simulink model "Thruster_Example_rw"  (R2024b)
settings: Solver=ode4  StartTime=0.0  StopTime=2000  FixedStep=0.01  RelTol=1e-3
undefined symbols (not defined in the file): Cube_L, dt, F_vec, Iws, M_rw, m_tot, norm_Ib, Omega1_init, Omega2_init, Omega3_init, Omega4_init, qb0, rad2rpm, RCS_F, RCS_F_vec, RCS_Pos, RCS_pos, RCS_PWM_Freq, RCS_Sampling_time, RCS_THR_vec, REL_TS_POS_I_0, REL_TS_VEL_I_0, RW_As, RW_Max_Speed, RW_Omegad_max, sat, SC_Ib, SC_state0, SS_Total_Mass, TC_Kepler, THR_dt, THR_Force, THR_freq, THR_Pos, TS_Ib, TS_qb0, TS_state0, TS_wb0, wb0, X, Y, Z
libraries: sm_lib x348, nesl_utility x236, simulink_extras x115, sharedtransform x64, aerolibutil x38, simulink x28, sharedutil x13
(part 16 of 16)

== matlab function Thruster_Example_rw/Prac1/Subsystem/Thruster Allocation ==
  settings: updateMethod=DISCRETE
  data: u_pwm output; F_B_cmd input; tau_B_cmd input; F_B_real output; tau_B_real output; r input; d input; F_max input
function [u_pwm, F_B_real, tau_B_real] = ALLOC_THRUSTER_PWM_16(F_B_cmd, tau_B_cmd, r, d, F_max)
%#codegen
% ============================================================
% Allocation block
% Input :
%   F_B_cmd    [3x1] desired total body force
%   tau_B_cmd  [3x1] desired total body torque
%
% Output:
%   u_pwm      [12x1] thruster duty command, 0 ~ 1
%   F_B_real   [3x1] realized body force after allocation
%   tau_B_real [3x1] realized body torque after allocation
%
% Example:
%   12-thruster layout for 6DoF control
%   Replace thruster geometry / Tmax below with your real spacecraft values.
% ============================================================

    % Build 6x12 thruster mapping matrix A
    A = build_thruster_matrix( 16, r, d, F_max);

    % Desired wrench
    w_cmd = [F_B_cmd; tau_B_cmd];

    % Bounded least-squares allocation: 0 <= u <= 1
    u_pwm = bounded_allocator_0_1(A, w_cmd);

    % Realized wrench
    w_real     = A * u_pwm;
    F_B_real   = w_real(1:3);
    tau_B_real = w_real(4:6);
end


% ============================================================
% Thruster layout
% ============================================================
function A = build_thruster_matrix(N, r, d, F_max)
    % --------------------------------------------------------
    % Example spacecraft half-size [m]
    % Replace with your real geometry
    % --------------------------------------------------------
    % L = 0.50;   % lever arm

    % --------------------------------------------------------
    % Max thrust of each thruster [N]
    % Replace with your real thruster max force
    % --------------------------------------------------------
    Tmax = F_max * ones(N,1);

    % --------------------------------------------------------
    % Thruster positions r_i in body frame [m]
    % Each column is one thruster position
    % --------------------------------------------------------
    % r = [ ...
    %      0,   0,   0,   0,   L,  -L,   L,  -L,   L,  -L,   L,  -L;
    %      L,  -L,   L,  -L,   0,   0,   0,   0,   L,   L,  -L,  -L;
    %      L,  -L,  -L,   L,   L,  -L,  -L,   L,   0,   0,   0,   0 ];

    % --------------------------------------------------------
    % Thruster unit directions d_i in body frame
    %
    % T1,T2 : +X
    % T3,T4 : -X
    % T5,T6 : +Y
    % T7,T8 : -Y
    % T9,T10: +Z
    % T11,T12:-Z
    % --------------------------------------------------------
    % d = [ ...
    %      1,   1,  -1,  -1,   0,   0,   0,   0,   0,   0,   0,   0;
    %      0,   0,   0,   0,   1,   1,  -1,  -1,   0,   0,   0,   0;
    %      0,   0,   0,   0,   0,   0,   0,   0,   1,   1,  -1,  -1 ];

    % --------------------------------------------------------
    % Build A = [F; tau], size 6x12
    % --------------------------------------------------------
    A = zeros(6,N);

    for i = 1:N
        f_i       = Tmax(i) * d(:,i);
        tau_i     = cross(r(:,i), f_i);
        A(:,i)    = [f_i; tau_i];
    end
end


% ============================================================
% Bounded allocator: 0 <= u <= 1
% Codegen-friendly fixed-size active-set style
% ============================================================
function u = bounded_allocator_0_1(A, w_cmd)
    N = 16;
    u = zeros(N,1);

    % free_mask(i)=true means this thruster is still free to solve
    free_mask = true(N,1);

    lambda = 1e-8;   % small damping

    for iter = 1:(N+1)

        % Residual after fixed/saturated thrusters
        w_res = w_cmd;
        for i = 1:N
            if ~free_mask(i)
                w_res = w_res - A(:,i) * u(i);
            end
        end

        % Collect free columns into Af (fixed-size construction)
        Af  = zeros(6,N);
        idx = zeros(N,1);
        nf  = 0;

        for i = 1:N
            if free_mask(i)
                nf = nf + 1;
                idx(nf) = i;
                Af(:,nf) = A(:,i);
            end
        end

        if nf == 0
            break;
        end

        % Minimum-norm damped solution on free set
        M       = Af * Af.' + lambda * eye(6);
        uf_full = Af.' * (M \ w_res);   % size Nx1, only first nf entries used

        % Put candidate solution into u
        for k = 1:nf
            i = idx(k);
            u(i) = uf_full(k);
        end

        % Check bounds and fix saturated variables
        violated = false;
        for k = 1:nf
            i = idx(k);

            if u(i) < 0
                u(i) = 0;
                free_mask(i) = false;
                violated = true;

            elseif u(i) > 1
                u(i) = 1;
                free_mask(i) = false;
                violated = true;
            end
        end

        if ~violated
            break;
        end
    end

    % Final clipping
    for i = 1:N
        if u(i) < 0
            u(i) = 0;
        elseif u(i) > 1
            u(i) = 1;
        end
    end
end

== matlab function Thruster_Example_rw/Prac1/TS 6-DOF Dynamics ==
  data: w input; x input; Ib input; wd output; T_ext input; F_ext input; xd output
function [wd, xd]  = eq_propagate(w, x, Ib, T_ext, F_ext)
% % 
% 출력 1: 위성 동체 좌표계 각가속도
% 출력 2: 관성좌표계 선가속도

%% Rotational Motion
% wd = [0 0 0]';
wd = inv(Ib)*(T_ext - cross(w, Ib*w));

%% Translational Motion


u  = 3.9860064e+14; % earth gravitional parameter
Re = 6378137;      % earth radius [m]

xd = zeros(size(x));

v1_i = x(4); % x1 = dx/dt
v2_i = x(5); % y1 = dy/dt
v3_i = x(6); % z1 = dz/dt
p1_i = x(1); % x
p2_i = x(2); % y
p3_i = x(3); % z

r=sqrt(p1_i^2+p2_i^2+p3_i^2);

% % %   Keplar Motion Equatnion
% % %  => r_dd + u/(r^3)r_ = 0 => r_dd = -u/(r^3)r_
xd(1) = v1_i;
xd(2) = v2_i;
xd(3) = v3_i;
xd(4) = -u*p1_i/(r^3) +  F_ext(1);
xd(5) = -u*p2_i/(r^3) +  F_ext(2);
xd(6) = -u*p3_i/(r^3) +  F_ext(3);

end

== matlab function Thruster_Example_rw/CMG_Gimbal_Angle_Control_Example/Subsystem/Gimbal_Angle_Controller[PID] ==
  data: angle_cmd input; angle_mea input; t_cmd output; rate_mea input; dt input
function t_cmd = fcn(angle_cmd, angle_mea, rate_mea, dt)

persistent I_save

if isempty(I_save)
    I_save = 0.0;
end

kp = 1.0;
kd = 2.0;
ki = 0.01;

ang_err = angle_cmd - angle_mea;
rate_err = 0-rate_mea;

t_cmd = kp*ang_err + kd*rate_err + ki*I_save;

I_save = I_save + ang_err*dt;


end

== matlab function Thruster_Example_rw/Prac1/command_generator ==
  settings: updateMethod=DISCRETE
  data: rel_p_cmd output; flag input; rel_v_cmd output; Kp_pos output; Kd_pos output
function [rel_p_cmd,rel_v_cmd,Kp_pos,Kd_pos]  = Mission_Supporter(flag)

if flag == 1
    rel_p_cmd = [5 0 0]';
    rel_v_cmd = [0 0 0]';
    Kp_pos = 0.3;
    Kd_pos = 17;    
else
    rel_p_cmd = [5 0 0]';
    rel_v_cmd = [0 0 0]';
    Kp_pos =   0.3;
    Kd_pos = 17.0;    
end


end

== matlab function Thruster_Example_rw/Prac1/saturation ==
  data: max_speed input; res output; Omega_mea input; torque_cmd input
function res  = saturation(max_speed, Omega_mea, torque_cmd)

Omega1_mea = Omega_mea(1);
Omega2_mea = Omega_mea(2);
Omega3_mea = Omega_mea(3);
Omega4_mea = Omega_mea(4);

if abs(Omega1_mea)> max_speed
    res1 = 0;
else
    res1 = torque_cmd(1);
end

if abs(Omega2_mea)>max_speed
    res2 = 0;
else
    res2 = torque_cmd(2);
end

if abs(Omega3_mea)>max_speed
    res3 = 0;
else
    res3 = torque_cmd(3);
end

if abs(Omega4_mea)>max_speed
    res4 = 0;
else
    res4 = torque_cmd(4);
end

res = [res1,res2,res3,res4]';

end

== matlab function Thruster_Example_rw/Prac1/Simple PD Control ==
  settings: updateMethod=DISCRETE
  data: q_err input; u output; w_err input; Kp_rw input; Kd_rw input; u_prev output
function [u, u_prev] = Att_PD_Control(q_err, w_err, Kp_rw, Kd_rw)

persistent I_save
persistent flg
persistent u_save

if isempty(flg)
    flg = 1;
    I_save = [0 0 0]';
    u_save = [0 0 0]';
end
 
K3 = 0.0*diag([1 1 1]);

q_e_v = [q_err(2), q_err(3), q_err(4)]';

u_prev = u_save;

u = (Kp_rw*q_e_v + Kd_rw*w_err + K3*I_save);

u_save = u;

I_save = I_save + (q_e_v*0.01);

end

== matlab function Thruster_Example_rw/Prac1/QP Opt ==
  settings: updateMethod=DISCRETE
  data: tau_des input; u_rw_cmd output; Omega_rw input; dt input; tau_body_cmd output; exitflag_out output; RW_max_speed input
function [u_rw_cmd, tau_body_cmd, exitflag_out] = RW4_QP_Controller(tau_des, Omega_rw, dt, RW_max_speed)
%#codegen
%
% 4-wheel Reaction Wheel QP controller
% tau_body = -A_rw * u_rw
%
% Inputs:
%   tau_des   [3x1] desired body torque
%   Omega_rw  [4x1] current wheel speeds [rad/s]
%   u_prev    [4x1] previous wheel torque command [N*m]
%   dt        scalar control period [s]
%
% Outputs:
%   u_rw_cmd     [4x1] wheel motor torque command
%   tau_body_cmd [3x1] actual body torque from RW
%   exitflag_out scalar

persistent u_save;

if isempty(u_save)
    u_save = [0 0 0 0]';
end

u_rw_cmd     = zeros(4,1);
tau_body_cmd = zeros(3,1);
exitflag_out = 0;

tau_des  = reshape(tau_des,  [3,1]);
Omega_rw = reshape(Omega_rw, [4,1]);
u_prev   = u_save;

% =========================
% RW axis matrix (3x4)
% =========================
A_rw = [0.70710678,  0.0,        -0.70710678,  0.0;
        0.0,         0.70710678,  0.0,        -0.70710678;
        0.70710678,  0.70710678,  0.70710678,  0.70710678 ];

% =========================
% User parameters
% =========================
% Torque tracking weight (body torque tracking)
Wtau = diag([10.0, 10.0, 10.0]);

% Wheel torque magnitude penalty
Wu = 1e-3 * eye(4);

% Wheel torque smoothing penalty
Wr = 1e-2 * eye(4);

% Optional wheel-speed centering penalty
% Start with very small values. Increase later if wheel speeds drift too much.
Wh = zeros(4,4);
Wh = 1e-6 * eye(4);
% 예: Wh = 1e-6 * eye(4);

% Wheel inertia about spin axis [kg*m^2]
Jw = 0.227*[1;1;1;1];

% Wheel torque limits [N*m]
u_max = [0.2; 0.2; 0.2; 0.2];
u_min = -u_max;

% Wheel torque rate limits [N*m/s]
du_max = [0.20; 0.20; 0.20; 0.20];
du_min = -du_max;

% Wheel speed limits [rad/s]
Omega_max = [RW_max_speed;RW_max_speed;RW_max_speed;RW_max_speed];
Omega_min = -Omega_max;

% =========================
% QP construction
%
% minimize 0.5*|| -A_rw*u - tau_des ||^2_Wtau
%        + 0.5*u'*Wu*u
%        + 0.5*(u-u_prev)'*Wr*(u-u_prev)
%        + 0.5*(Omega_next)'*Wh*(Omega_next)
%
% Omega_next = Omega_rw + D*u
% D = diag(dt./Jw)
% =========================

D = diag(dt ./ Jw);

H = A_rw' * Wtau * A_rw + Wu + Wr + D' * Wh * D;
f = A_rw' * Wtau * tau_des - Wr * u_prev + D' * Wh * Omega_rw;

% Make H numerically symmetric
H = 0.5 * (H + H');

% =========================
% Constraints
% 1) wheel torque bounds
% 2) wheel torque rate bounds
% 3) next-step wheel speed bounds
% =========================

% Torque-rate bounds
lb_rate = u_prev + du_min * dt;
ub_rate = u_prev + du_max * dt;

% Speed-next bounds
% Omega_next = Omega_rw + dt*(u./Jw)
% => u >= Jw .* (Omega_min - Omega_rw)/dt
% => u <= Jw .* (Omega_max - Omega_rw)/dt
lb_speed = Jw .* ((Omega_min - Omega_rw) / dt);
ub_speed = Jw .* ((Omega_max - Omega_rw) / dt);

% Final bounds
lb = max(u_min, max(lb_rate, lb_speed));
ub = min(u_max, min(ub_rate, ub_speed));

% Feasibility repair
for i = 1:4
    if lb(i) > ub(i)
        c = 0.5 * (lb(i) + ub(i));
        lb(i) = c;
        ub(i) = c;
    end
end

% Empty linear inequality/equality constraints
A   = zeros(0,4);
b   = zeros(0,1);
Aeq = zeros(0,4);
beq = zeros(0,1);

% Initial guess for active-set
x0 = min(max(u_prev, lb), ub);

% quadprog codegen-friendly option
options = optimoptions('quadprog', ...
    'Algorithm', 'active-set', ...
    'ConstraintTolerance', 1e-6, ...
    'OptimalityTolerance', 1e-6, ...
    'StepTolerance', 1e-12, ...
    'MaxIterations', 50);

[u_sol, ~, exitflag] = quadprog(H, f, A, b, Aeq, beq, lb, ub, x0, options);

if exitflag <= 0 || isempty(u_sol)
    u_rw_cmd = x0;
else
    u_rw_cmd = u_sol;
end

tau_body_cmd = -A_rw * u_rw_cmd;
u_save = u_rw_cmd;
exitflag_out = exitflag;

== matlab function Thruster_Example_rw/Prac1/Subsystem/Get LOS Quaternion7 ==
  settings: updateMethod=DISCRETE
  data: r_rel input; v_rel input; r_ref input; v_ref input; a_ref input; q input; q_err input; w_err input; F_cmd_B output; tau_cmd_B output; m_sc input; Kp_pos input; Kd_pos input; Kp_att input; Kd_att input; r_err output; v_err output; q output; q_err_vec output; w_err output; a_cmd output
function [F_cmd_B, tau_cmd_B, r_err, v_err, q, q_err_vec, w_err, a_cmd] = ...
    relative_position_los_controller( ...
    r_rel, v_rel, ...          % [3x1] relative position/velocity
    r_ref, v_ref, a_ref, ...   % [3x1] desired relative pos/vel/acc
    q, q_err, w_err, ...                  % [4x1], [3x1] current attitude/angular velocity
    m_sc, Kp_pos, Kd_pos, Kp_att, Kd_att)
%#codegen
%
% q, q_los_ref : scalar-first quaternion [qw qx qy qz]'
%                body -> reference
% r_rel, r_ref, v_rel, v_ref, a_ref : reference frame 기준
%
% 출력:
% F_cmd_B   : [3x1] body frame force command
% tau_cmd_B : [3x1] body frame torque command

    F_cmd_B   = zeros(3,1);
    tau_cmd_B = zeros(3,1);
    r_err     = zeros(3,1);
    v_err     = zeros(3,1);
    q_err_vec = zeros(3,1);
    % w_err     = zeros(3,1);
    a_cmd     = zeros(3,1);

    %% 1) Relative position controller
    r_err = r_ref - r_rel;
    v_err = v_ref - v_rel;

    a_cmd = a_ref + Kp_pos * r_err + Kd_pos * v_err;
    F_cmd_R = m_sc * a_cmd;

    %% 2) Reference frame -> body frame
    % q : body -> reference
    % therefore F_B = C_BR' * F_R
    C_BR   = quat_to_dcm_sf(q);
    F_cmd_B = C_BR' * F_cmd_R;

    %% 3) LOS attitude controller

    % shortest path
    if q_err(1) < 0
        q_err = -q_err;
    end

    q_err_vec = q_err(2:4);

    tau_cmd_B = Kp_att * q_err_vec + Kd_att * w_err;
end


function q_out = quat_mul_sf(a, b)
% scalar-first quaternion multiplication
    q_out = [ a(1)*b(1) - a(2)*b(2) - a(3)*b(3) - a(4)*b(4);
              a(1)*b(2) + a(2)*b(1) + a(3)*b(4) - a(4)*b(3);
              a(1)*b(3) - a(2)*b(4) + a(3)*b(1) + a(4)*b(2);
              a(1)*b(4) + a(2)*b(3) - a(3)*b(2) + a(4)*b(1) ];
end


function C = quat_to_dcm_sf(q)
% scalar-first quaternion, body -> reference
    q = q / (sqrt(sum(q.^2)) + 1e-12);

    qw = q(1);
    qx = q(2);
    qy = q(3);
    qz = q(4);

    C = [1-2*(qy*qy+qz*qz),   2*(qx*qy-qw*qz),   2*(qx*qz+qw*qy);
         2*(qx*qy+qw*qz),     1-2*(qx*qx+qz*qz), 2*(qy*qz-qw*qx);
         2*(qx*qz-qw*qy),     2*(qy*qz+qw*qx),   1-2*(qx*qx+qy*qy)];
end

== matlab function Thruster_Example_rw/Prac1/Subsystem/Subsystem1/MinOnTime_Enforcer1 ==
  settings: updateMethod=DISCRETE
  data: relay_raw input; F_gated output; t input
function F_gated = fcn(relay_raw, t)
%#codegen
% 최소 ON 시간 강제기 (MIB 기반)
% t_min_on = 0.0700 s (70 ms)
persistent t_on_start was_on;
if isempty(was_on)
    was_on     = false;
    t_on_start = 0;
end
t_min_on = 0.0700;
if relay_raw == 1 && ~was_on
    t_on_start = t;
end
if relay_raw == 1
    F_gated = 1;
elseif was_on && (t - t_on_start) < t_min_on
    F_gated = 1;   % 아직 70ms 안 됐으면 강제 ON 유지
else
    F_gated = 0;
end
was_on = (F_gated == 1);

end

== matlab function Thruster_Example_rw/Prac1/Subsystem/Subsystem2/MinOnTime_Enforcer1 ==
  settings: updateMethod=DISCRETE
  data: relay_raw input; F_gated output; t input
function F_gated = fcn(relay_raw, t)
%#codegen
% 최소 ON 시간 강제기 (MIB 기반)
% t_min_on = 0.0700 s (70 ms)
persistent t_on_start was_on;
if isempty(was_on)
    was_on     = false;
    t_on_start = 0;
end
t_min_on = 0.0700;
if relay_raw == 1 && ~was_on
    t_on_start = t;
end
if relay_raw == 1
    F_gated = 1;
elseif was_on && (t - t_on_start) < t_min_on
    F_gated = 1;   % 아직 70ms 안 됐으면 강제 ON 유지
else
    F_gated = 0;
end
was_on = (F_gated == 1);

end

== matlab function Thruster_Example_rw/Prac1/Subsystem/Subsystem3/MinOnTime_Enforcer1 ==
  settings: updateMethod=DISCRETE
  data: relay_raw input; F_gated output; t input
function F_gated = fcn(relay_raw, t)
%#codegen
% 최소 ON 시간 강제기 (MIB 기반)
% t_min_on = 0.0700 s (70 ms)
persistent t_on_start was_on;
if isempty(was_on)
    was_on     = false;
    t_on_start = 0;
end
t_min_on = 0.0700;
if relay_raw == 1 && ~was_on
    t_on_start = t;
end
if relay_raw == 1
    F_gated = 1;
elseif was_on && (t - t_on_start) < t_min_on
    F_gated = 1;   % 아직 70ms 안 됐으면 강제 ON 유지
else
    F_gated = 0;
end
was_on = (F_gated == 1);

end

== matlab function Thruster_Example_rw/rigid body/rigid body1 ==
  data: w input; q_prime output; q input
function q_prime = fcn(w,q)

F_q = (1/2)*[0 -w(1) -w(2) -w(3);
       w(1) 0 w(3) -w(2);
       w(2) -w(3) 0 w(1);
       w(3) w(2) -w(1) 0];

q_prime = F_q*q;

== matlab function Thruster_Example_rw/Prac1/Subsystem/Subsystem4/MinOnTime_Enforcer1 ==
  settings: updateMethod=DISCRETE
  data: relay_raw input; F_gated output; t input
function F_gated = fcn(relay_raw, t)
%#codegen
% 최소 ON 시간 강제기 (MIB 기반)
% t_min_on = 0.0700 s (70 ms)
persistent t_on_start was_on;
if isempty(was_on)
    was_on     = false;
    t_on_start = 0;
end
t_min_on = 0.0700;
if relay_raw == 1 && ~was_on
    t_on_start = t;
end
if relay_raw == 1
    F_gated = 1;
elseif was_on && (t - t_on_start) < t_min_on
    F_gated = 1;   % 아직 70ms 안 됐으면 강제 ON 유지
else
    F_gated = 0;
end
was_on = (F_gated == 1);

end

== matlab function Thruster_Example_rw/Prac1/Subsystem/Subsystem5/MinOnTime_Enforcer1 ==
  settings: updateMethod=DISCRETE
  data: relay_raw input; F_gated output; t input
function F_gated = fcn(relay_raw, t)
%#codegen
% 최소 ON 시간 강제기 (MIB 기반)
% t_min_on = 0.0700 s (70 ms)
persistent t_on_start was_on;
if isempty(was_on)
    was_on     = false;
    t_on_start = 0;
end
t_min_on = 0.0700;
if relay_raw == 1 && ~was_on
    t_on_start = t;
end
if relay_raw == 1
    F_gated = 1;
elseif was_on && (t - t_on_start) < t_min_on
    F_gated = 1;   % 아직 70ms 안 됐으면 강제 ON 유지
else
    F_gated = 0;
end
was_on = (F_gated == 1);

end

== matlab function Thruster_Example_rw/Prac1/Subsystem/Subsystem6/MinOnTime_Enforcer1 ==
  settings: updateMethod=DISCRETE
  data: relay_raw input; F_gated output; t input
function F_gated = fcn(relay_raw, t)
%#codegen
% 최소 ON 시간 강제기 (MIB 기반)
% t_min_on = 0.0700 s (70 ms)
persistent t_on_start was_on;
if isempty(was_on)
    was_on     = false;
    t_on_start = 0;
end
t_min_on = 0.0700;
if relay_raw == 1 && ~was_on
    t_on_start = t;
end
if relay_raw == 1
    F_gated = 1;
elseif was_on && (t - t_on_start) < t_min_on
    F_gated = 1;   % 아직 70ms 안 됐으면 강제 ON 유지
else
    F_gated = 0;
end
was_on = (F_gated == 1);

end

== matlab function Thruster_Example_rw/Prac1/Subsystem/Subsystem7/MinOnTime_Enforcer1 ==
  settings: updateMethod=DISCRETE
  data: relay_raw input; F_gated output; t input
function F_gated = fcn(relay_raw, t)
%#codegen
% 최소 ON 시간 강제기 (MIB 기반)
% t_min_on = 0.0700 s (70 ms)
persistent t_on_start was_on;
if isempty(was_on)
    was_on     = false;
    t_on_start = 0;
end
t_min_on = 0.0700;
if relay_raw == 1 && ~was_on
    t_on_start = t;
end
if relay_raw == 1
    F_gated = 1;
elseif was_on && (t - t_on_start) < t_min_on
    F_gated = 1;   % 아직 70ms 안 됐으면 강제 ON 유지
else
    F_gated = 0;
end
was_on = (F_gated == 1);

end

== matlab function Thruster_Example_rw/Prac1/Subsystem/Subsystem8/MinOnTime_Enforcer1 ==
  settings: updateMethod=DISCRETE
  data: relay_raw input; F_gated output; t input
function F_gated = fcn(relay_raw, t)
%#codegen
% 최소 ON 시간 강제기 (MIB 기반)
% t_min_on = 0.0700 s (70 ms)
persistent t_on_start was_on;
if isempty(was_on)
    was_on     = false;
    t_on_start = 0;
end
t_min_on = 0.0700;
if relay_raw == 1 && ~was_on
    t_on_start = t;
end
if relay_raw == 1
    F_gated = 1;
elseif was_on && (t - t_on_start) < t_min_on
    F_gated = 1;   % 아직 70ms 안 됐으면 강제 ON 유지
else
    F_gated = 0;
end
was_on = (F_gated == 1);

end

== matlab function Thruster_Example_rw/Prac1/Subsystem/RCS_Relative_Position_Control_Allocation1 ==
  settings: updateMethod=DISCRETE
  data: F_cmd input; tau_cmd input; RCS_pos input; RCS_F_vec input; Tmax input; duty output; F_est output; tau_est output; F_err output; tau_err output; sat_ratio output; wF input; wT input
function [duty, F_est, tau_est, F_err, tau_err, sat_ratio] = ...
    rcs_force_torque_allocator(F_cmd, tau_cmd, RCS_pos, RCS_F_vec, Tmax, wF, wT)
%#codegen
%
% F_cmd      : [3x1] commanded force in body frame [N]
% tau_cmd    : [3x1] commanded torque in body frame [N*m]
% RCS_pos    : [3xN] thruster positions in body frame [m]
% RCS_F_vec  : [3xN] thruster direction vectors
% Tmax       : scalar, max thrust of one thruster [N]
% wF         : scalar, force tracking weight
% wT         : scalar, torque tracking weight
%
% duty       : [N x 1], 0~1
% F_est      : [3x1], achieved force [N]
% tau_est    : [3x1], achieved torque [N*m]
% F_err      : [3x1], force error [N]
% tau_err    : [3x1], torque error [N*m]
% sat_ratio  : saturated thruster ratio

    N = size(RCS_pos, 2);

    duty      = zeros(N,1);
    F_est     = zeros(3,1);
    tau_est   = zeros(3,1);
    F_err     = zeros(3,1);
    tau_err   = zeros(3,1);
    sat_ratio = 0;

    Fmat = zeros(3, N);
    Tmat = zeros(3, N);

    for i = 1:N
        dir_i = RCS_F_vec(:,i);
        nrm   = sqrt(sum(dir_i.^2));

        if nrm > 1e-12
            dir_i = dir_i / nrm;
        else
            dir_i = [0;0;0];
        end

        Fi = Tmax * dir_i;
        Ti = cross3(RCS_pos(:,i), Fi);

        Fmat(:,i) = Fi;
        Tmat(:,i) = Ti;
    end

    % Solve:
    % min || wF*(Fmat*u - F_cmd) ||^2 + || wT*(Tmat*u - tau_cmd) ||^2
    % s.t. 0 <= u <= 1

    A = [wF * Fmat;
         wT * Tmat];

    b = [wF * F_cmd;
         wT * tau_cmd];

    H = A' * A + 1e-8 * eye(N);
    g = A' * b;

    alpha = 1.0 / (trace(H) + 1e-9);
    u = zeros(N,1);

    for k = 1:150
        grad = H * u - g;
        u    = u - alpha * grad;

        for j = 1:N
            if u(j) < 0
                u(j) = 0;
            elseif u(j) > 1
                u(j) = 1;
            end
        end
    end

    duty    = u;
    F_est   = Fmat * duty;
    tau_est = Tmat * duty;

    F_err   = F_cmd   - F_est;
    tau_err = tau_cmd - tau_est;

    sat_ratio = sum(duty > 0.999) / N;
end


function c = cross3(a, b)
    c = [ a(2)*b(3) - a(3)*b(2);
          a(3)*b(1) - a(1)*b(3);
          a(1)*b(2) - a(2)*b(1) ];
end

== matlab function Thruster_Example_rw/Prac1/SS Attitude Control wrt ECI ==
  settings: updateMethod=DISCRETE
  data: q_err input; RW_cmd output; w_err input; As input; Kp_rw input; Kd_rw input
function RW_cmd  = Att_PD_Control(q_err, w_err, As,Kp_rw,Kd_rw)

persistent I_save
persistent flg

if isempty(flg)
    flg = 1;
    I_save = [0 0 0]';
end
 
K3 = 0.0*diag([1 1 1]);

q_e_v = [q_err(2), q_err(3), q_err(4)]';

u = Kp_rw*q_e_v + Kd_rw*w_err + K3*I_save;

RW_cmd = pinv(As)*-u;

I_save = I_save + (q_e_v*0.01);

end

== matlab function Thruster_Example_rw/rigid body/rigid body2 ==
  data: angle output; q input
function angle = quat2eulang(q)
% ZYX 회전 가정

% q0 = q(1); q1 = q(2); q2 = q(3); q3 = q(4);
% 
% yaw = atan2(2*(q1*q2 + q0*q3), q0^2+q1^2-q2^2-q3^2);
% 
% s = 2*(q0*q2 - q3*q1);
% s = max(-1, min(1, s));      % clamp
% pitch = asin(s);
% 
% roll = atan2(2*(q2*q3 + q0*q1), q0^2-q1^2-q2^2+q3^2);



% % 'ZYX' 회전에서 DCM을 Body-frame -> 관성좌표계 으로 정의할 때, 각을 구하는 상황.
% % /                cos(psi) cos(theta),                              cos(theta) sin(psi),                   -sin(theta)     \
% % |                                                                                                                         |
% % | cos(psi) sin(phi) sin(theta) - cos(phi) sin(psi), cos(phi) cos(psi) + sin(phi) sin(psi) sin(theta), cos(theta) sin(phi) |
% % |                                                                                                                         |
% % \ sin(phi) sin(psi) + cos(phi) cos(psi) sin(theta), cos(phi) sin(psi) sin(theta) - cos(psi) sin(phi), cos(phi) cos(theta) /
R = quat2DCM(q);
yaw   = atan2(R(1,2), R(1,1));
pitch = -asin(R(1,3));
roll  = atan2(R(2,3), R(3,3));



% angle = [roll, pitch, yaw]';
angle = [yaw, pitch, roll]'; %MATLAB 에서는 [roll, pitch, yaw] 가 아닌 [yaw, pitch, roll] 순으로 값을 반환한다.
% 실제 도움말을 보면, 반환각 벡터에 대해 "Ψ is R1, Θ is R2, and Φ is R3." 으로 나와있는 것을 볼 수 있다.



function R = quat2DCM(q)

q0 = q(1); q1 = q(2); q2 = q(3); q3 = q(4);

%% DCM을 관성좌표계 -> Body-frame 으로 정의할 때의 행렬 
% R = [2*(q0^2 + q1^2)-1, 2*(q1*q2 - q0*q3),2*(q1*q3 + q2*q0);
%      2*(q1*q2 + q0*q3), 2*(q0^2 + q2^2)-1, 2*(q2*q3 - q1*q0);
%      2*(q1*q3 - q2*q0), 2*(q2*q3 + q1*q0), 2*(q0^2 + q3^2)-1];

%% DCM을 Body-frame -> 관성좌표계 으로 정의할 때의 행렬 
R = [q0^2+q1^2-q2^2-q3^2, 2*(q1*q2 + q0*q3), 2*(q1*q3 - q2*q0);
     2*(q1*q2 - q0*q3), q0^2-q1^2+q2^2-q3^2, 2*(q2*q3 + q1*q0);
     2*(q1*q3 + q2*q0), 2*(q2*q3 - q1*q0), q0^2-q1^2-q2^2+q3^2];

end

end

== matlab function Thruster_Example_rw/Reaction_Wheel_Simple1/rigid body ==
  data: t_ext input; omega_prime output; omega input; omega_rw input; omega_rw_prime input
% function omega_prime = fcn(t_ext, omega,u)
function omega_prime = fcn(t_ext, omega,omega_rw,omega_rw_prime)
% function omega_prime = fcn(Ib,t_ext, omega,omega_rw,omega_rw_prime)
L = [0.3 0.3 0.3]'; %Length([m]) of cube 
M = 10; %Mass([kg]) of cube

R=0.015; % Radius([m]) of cylinder(Reaction wheel)
M_rw=0.01; % Mass([kg]) of cylinder(Reaction wheel)
L_rw=0.01; % Length([m]) of cylinder(Reaction wheel)

% Density([kg/m^3]) of cube
density = M/(L(1)*L(2)*L(3));   
% MOI([kg*m^2]) of cube
I = [ 1/12*M*(L(2)^2+L(3)^2) 0 0;
      0 1/12*M*(L(1)^2+L(3)^2) 0;
      0 0 1/12*M*(L(1)^2+L(2)^2)];

% MOI([kg*m^2]) of cylinder(Reaction wheel)
I_rw=[1/4*M_rw*R^2+1/12*M_rw*L_rw^2 0 0;
    0 1/4*M_rw*R^2+1/12*M_rw*L_rw^2 0;
    0 0 1/2*M_rw*R^2];

Ib = I; % body's MOI should include whole MOI.
        % No!! Ib is just cube's MOI!!

%control input torque
% u=-(I_rw*omega_rw_prime+cross(omega,I_rw*omega_rw));
u=I_rw*omega_rw_prime+cross(omega,I_rw*omega_rw);

% omega_prime = inv(Ib)*(t_ext+u - cross(omega,Ib*omega));
omega_prime = inv(Ib)*(t_ext-u - cross(omega,Ib*omega));
% control intput "u" has opposite direction with "t_ext"

== matlab function Thruster_Example_rw/rigid body/Att Kinematic1 ==
  data: ang input; w input; ang_prime output
function ang_prime = fcn(ang,w)

phi = ang(1);   %roll
theta = ang(2); %pitch
psi = ang(3);   %yaw

Att = [1 sin(phi)*tan(theta) cos(phi)*tan(theta);
    0 cos(phi) -sin(phi);
    0 sin(phi)*sec(theta) cos(phi)*sec(theta)];

ang_prime = Att*w;
